simulink model "PPS_Scenario_003_cs"  (Simulink 7.6)
settings: Solver=ode5  SolverMode=SingleTasking  StartTime=0.0  StopTime=inf  FixedStep=1/100  RelTol=1e-3
PreLoadFcn:
  | check_NUTS_defined;
  | 
  | assignin('base',['model_closed_' bdroot],false);
  | 
  | addpath('../includes_PPS');
  | 
  | if exist('PPS_Model_sfun.mexw64')==3
  | delete PPS_Model_sfun.mexw64;
  | end
  | 
  | if exist('PPS_Model_sfun.mexw32') ==3
  | delete PPS_Model_sfun.mexw32;
  | end
  | 
  | switch version('-release')
  | case {'2010a', '2010b', '2011a'}
  | addpath('../includes_PPS/ML2010a');
  | case {'2011b', '2012a', '2012b'}
  | addpath('../includes_PPS/ML2011b');
  | otherwise
  | addpath('../includes_PPS/ML2011b');
  | end
InitFcn:
  | PreScanExperimentInitFcn(bdroot)
StopFcn:
  | PreScanExperimentStopFcn(bdroot)
undefined symbols (not defined in the file): DiscIntNeverNeededParam, InitImageOutputDir, x_ini_VRML, y_ini_VRML, z_ini_VRML
libraries: PreScanSimulinkLibrary x48, simulink x27, PreScanUsefulBlocks x20, simulink_extras x9, simulink_need_slupdate x1
(part 2 of 14)

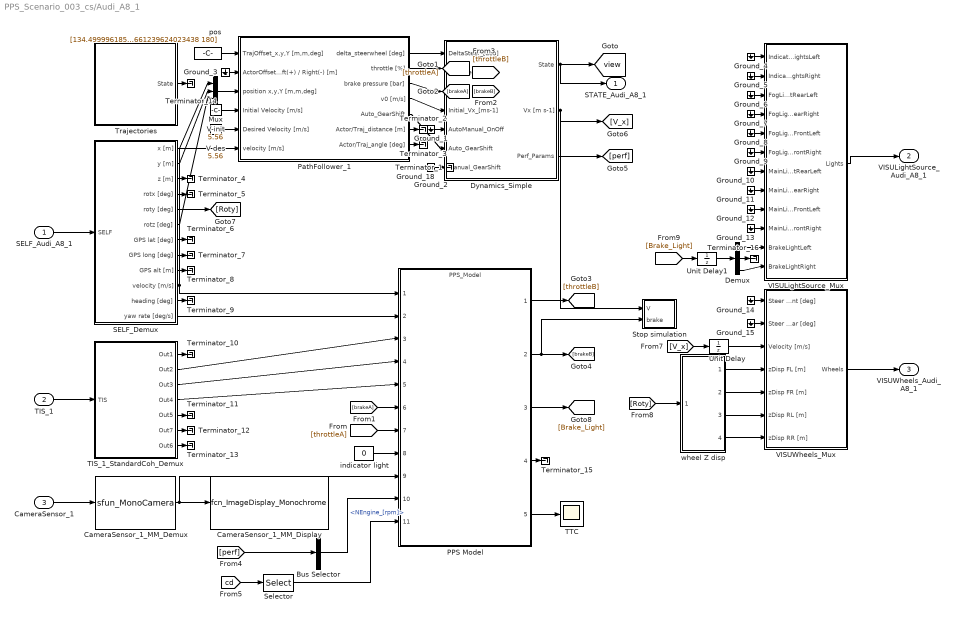
== system PPS_Scenario_003_cs/Audi_A8_1 ==
  SELF_Audi_A8_1 : Inport  Tag=SELFInport
  TIS_1 : Inport  Tag=RadarInport  Port=2  OutDataTypeStr=Bus: PRESCAN_SCANNERSENSORMESSAGE
  CameraSensor_1 : Inport  Tag=CameraSensorInport  Port=3  SampleTime=1/50
  Bus Selector : BusSelector  OutputSignals=NEngine_[rpm]
  CameraSensor_1_MM_Demux : S-Function  Tag=CameraSensor_Monochrome_Demux  FunctionName=sfun_MonoCamera  Parameters=[VerticalResolution HorizontalResolution] FrameRate SensorName CameraType SharedMemTag SharedMemRightTag DataType HasInputPort  EnableBusSupport=off  mask{HorizontalResolution=500, VerticalResolution=375, FrameRate=50, SensorName=CameraSensor_1, CameraType=Mono, SharedMemTag=CameraSensor_1_monoBeam_viewer_RGB, SharedMemRightTag=CameraSensor_1_StereoRight_viewer_RGB, DataType=uint8, HasInputPort=1}
      mask prompts: HorizontalResolution "User Specified: Horizontal Resolution [pixels]"; VerticalResolution "User Specified: Vertical Resolution [pixels]"; FrameRate "User Specified: Frame Rate [Hz]"; SensorName "User Specified: Camera Sensor Name"; CameraType "Camera type"; SharedMemTag "Tag for shared memory for main img"; SharedMemRightTag "Tag for shared memory for right img"; DataType "Image data type"; HasInputPort "Has input port"
      mask init:
      | if CameraType==1
      |     CameraTypeName='MONO';
      |     CameraPort1Name='I';
      |     CameraPort2Name='I';
      |     PortNumber=0;
      | else
      |     CameraTypeName='STEREO';
      |     CameraPort1Name='Left';
      |     CameraPort2Name='Right';
      |     PortNumber=1;
      | end
      settings: DeleteFcn=PreScanBlockDeleteFcn;
      mask StyleString: edit,edit,edit,edit,popup(Mono|Stereo),edit,edit,popup(uint8|single),edit
      mask Display:
      | fprintf('%s CAMERA:\n Monochrome\n%s \n V: %d x %d \n %d fps',CameraTypeName,SensorName,VerticalResolution,HorizontalResolution,FrameRate)
      | port_label('output',1,CameraPort1Name)
      | port_label('output',PortNumber+1,CameraPort2Name)
  CameraSensor_1_MM_Display : M-S-Function  Tag=CameraSensor_Monochrome_Display  InitFcn=InitImageOutputDir(gcb);  FunctionName=fcn_ImageDisplay_Monochrome  Parameters=SensorName EnableDisplay EnablePosition DisplayPosition FigureHandle SaveResults BitmapFormat TempOutputDir CameraType DataType  mask(PreScan Monochrome Display Block){SensorName=CameraSensor_1, EnableDisplay=on, EnablePosition=off, DisplayPosition=[10 10 500 375], FigureHandle=700, SaveResults=off, Format=PNG, TempOutputDir=0, CameraType=Mono, DataType=uint8}
      mask prompts: SensorName "User Specified: Title of Display"; EnableDisplay "Active"; EnablePosition "Set Display window position"; DisplayPosition "Display window position [xpos ypos width height]"; FigureHandle "Unique handle"; SaveResults "Save results"; TempOutputDir "OutputDir"; CameraType "Camera Type"; DataType "Image Data Type"
      mask help: This block displays the Monochrome output of a PreScan camera sensor.
      mask init:
      | if EnableDisplay
      |     EnableString='';
      |     EnableColor='gray';
      | else
      |     EnableString='INACTIVE';
      |     EnableColor='red';
      | end
      | switch Format
      |     case 1
      |         BitmapFormat = 'png';
      |     case 2
      |         BitmapFormat = 'bmp';
      |     case 3
      |         BitmapFormat = 'jpg';
      | end
      | if CameraType==1
      |     CameraTypeName='MONO';
      |     PortNumber=0;
      | else
      |     CameraTypeName='STEREO';
      |     PortNumber=1;
      | end
      settings: CopyFcn=CopyFcnDisplay  DeleteFcn=PreScanBlockDeleteFcn;  ModelCloseFcn=fcn_ImageDisplay_ModelCloseFcn
      mask Help: eval('openHelp(457)')
      mask StyleString: edit,checkbox,checkbox,edit,edit,checkbox,popup(PNG|BMP|JPG),edit,popup(Mono|Stereo),popup(uint8|single)
      mask CallbackString:
      | ||MV=get_param(gcb,'MaskVisibilities');
      | if strcmp(get_param(gcb,'EnablePosition'),'on')
      |     MV{4}='on';
      | else
      |     MV{4}='off';
      | end
      | set_param(gcb,'MaskVisibilities',MV);|||||||
      mask Display:
      | color(EnableColor);
      | fprintf('%s\n DISPLAY:\n Monochrome\n %s',EnableString,SensorName)
      | port_label('input',1,'I')
      | port_label('input',PortNumber+1,'I')
  Demux : Demux  Outputs=3
  Dynamics_Simple : Subsystem  Tag=Simple_Vehicle_Dynamics  mask(PreScan Block: Simple Dynamics){Migrate=off, TimeStep=1/100, ComputationMode=Continuous_Time}
      mask prompts: Migrate "Migrate. During migration this block will be replaced by a newer one."; TimeStep "Auto assigned: Time Step [s]"; ComputationMode "Computation mode:"
      mask help:
      | The Simple Dynamics Model is selected in the GUI to simulate vehicle dynamics behavior.
      |
      | The Simple Dynamics Model is completely open to the user. The parameters of this model can be set in the Simple Dynamics dialog in the GUI.
      |
      | For more information, please click Help.
      mask init:
      | p = SimpleDyn_pars;
      settings: DeleteFcn=PreScanBlockDeleteFcn;
      mask Help: eval('openHelp(220)')
      mask Display:
      | image(imread('SimpleDyn.png'))
      | port_label('input', 1, '{\delta}_S_t_ _e_e_r [deg]','texmode','on')
      | port_label('input', 2, 'Throttle [%]')
      | port_label('input', 3, 'Brake Pres [bar]')
      | port_label('input', 4, 'V_0 [ms-1]','texmode','on')
      | port_label('input', 5, 'Auto=[0]/Manual=[1]')
      | port_label('input', 6, 'Auto_GearShift')
      | port_label('input', 7, 'Manual_GearShift')
      | port_label('output', 1, 'State')
      | port_label('output', 2, 'Vx [ms-1]')
      | port_label('output', 3, 'Perf Params')
  Ground_{1..15,18} (16 alike) : Ground
  Mux : Mux  Inputs=3
  PPS Model : ModelReference  StopFcn=|  ModelNameDialog=PPS_Model  SimulationMode=Normal  ModelReferenceVersion=1.1238  CopyOfModelName=PPS_Model
      | if VRU_DisplaySwitch
      | CSpanel = findobj('Tag','cs_panel');
      | CSvalue = findobj('Tag','cs_value');
      | if VRU_EGO_State_Coll
      |    % Collision occured
      | %	bname = find_system('Tag', 'test num');	% get block name
      | %	test_num = mod( str2num(get_param(bname{:},'Value')), 5 );	% get block value
      | %	vel = ( test_num )*10+10;	% velocity
      |    set(CSpanel, 'BorderWidth',2, 'ForegroundColor',[0 120/255 0], 'HighlightColor',[0 120/255 0], 'ShadowColor', [0 120/255 0]);
      |    set(CSvalue, 'ForegroundColor',[0 120/255 0], 'String', strcat('Speed reduction', sprintf( ' %.1f ',VRU_EGO_State_BrakeVel-VRU_EGO_State_Coll), ' km/h'));
      |    set(CSpanel, 'Visible', 'On');
      |    set(CSvalue, 'Visible', 'On');
      | else
      |     if VRU_EGO_State_Flag06
      |         % Collision almost occur
      | 	set(CSpanel, 'BorderWidth',2, 'ForegroundColor','Green', 'HighlightColor','Green', 'ShadowColor', 'Green');
      | 	set(CSvalue, 'ForegroundColor','Green', 'String', 'Collision avoided');
      |         set(CSpanel, 'Visible', 'On');
      |         set(CSvalue, 'Visible', 'On');
      |     else
      |         % No risk of collision
      | 	set(CSpanel, 'Visible', 'Off');
      |         set(CSvalue, 'Visible', 'Off');
      |     end
      | end
      | clear CSpanel CSvalue VRU_EGO_State_Flag06 VRU_EGO_State_BrakeVel
      | end
      | PPS_Speed_Profile(VRU_simout,VRU_EGO_State_Coll);
      | PPS_TTC_Profile(VRU_simout,VRU_EGO_State_Coll);
  PathFollower_1 : Subsystem  Tag=pathFollower  mask(PreScan Block: Path Follower){Migrate=on, FileName='Car_trajectory_1.mat', TunableSteeringGain=1, XShifting_wrt_COG=0}
      mask prompts: Migrate "Migrate. During migration this block will be replaced by a newer one."; FileName "Trajectory Name"; TunableSteeringGain "TunableSteeringGain [-]"; XShifting_wrt_COG "XShifting_wrt_COG [m]"
      mask help:
      | The Path Follower Model is selected in the GUI to simulate driver behavior.
      |
      | For more information, please click Help.
      mask init:
      | load(['trajectories/',eval(FileName)])
      | traject=trajectory';
      | 
      | Traj_x=traject(:,2);
      | Traj_y=traject(:,3);
      | Traj_z=traject(:,4);
      | Traj_vx=traject(:,8);
      | Traj_vy=traject(:,9);
      | Traj_vz=traject(:,10);
      mask Help: eval('openHelp(232)')
  SELF_Demux : Subsystem  Tag=DemuxSELF
      settings: DeleteFcn=PreScanBlockDeleteFcn;
      mask Type: PreScan Demux Block:
      mask Display:
      | port_label('output',1,'x [m]')
      | port_label('output',2,'y [m]')
      | port_label('output',3,'z [m]','texmode','on')
      | port_label('output',4,'Rotx [deg]','texmode','on')
      | port_label('output',5,'Roty [deg]','texmode','on')
      | port_label('output',6,'Rotz [deg]','texmode','on')
      | port_label('output',7,'GPS lat [deg]','texmode','on')
      | port_label('output',8,'GPS long [deg]','texmode','on')
      | port_label('output',9,'GPS alt [m]','texmode','on')
      | port_label('output',10,'Velocity [m/s]')
      | port_label('output',11,'Heading [deg]')
      | port_label('output',12,'Yaw rate [deg/s]')
  Selector : Selector  InputPortWidth=5  IndexOptions=Index vector (dialog)  Indices=1  OutputSizes=1
  Stop simulation : Subsystem
  TIS_1_StandardCoh_Demux : Subsystem  TreatAsAtomicUnit=on  mask(PreScan Demux Block: TIS){MAXMESSAGES=32}
      mask prompts: MAXMESSAGES "Number of Objects"
      mask Help: eval('openHelp(441)')
      mask Display:
      | port_label('input',1,'TIS')
      | port_label('output',1,'Beam ID [-]')
      | port_label('output',2,'Range [m]')
      | port_label('output',3,'DopplerVelocity [m/s]')
      | port_label('output',4,'{\theta} [deg]','texmode','on')
      | port_label('output',5,'{\phi} [deg]','texmode','on')
      | port_label('output',6,'Target ID [-]','texmode','on')
      | port_label('output',7,'TIS Data','texmode','on')
  TTC : Scope
      settings: TimeRange=4.5  YMin=8  YMax=15
  Terminator_{1..16} (16 alike) : Terminator
  Trajectories : Subsystem  Tag=Trajectories
      settings: DeleteFcn=PreScanBlockDeleteFcn;
      mask Type: PreScan Source Block: Trajectories
      mask Description:
      | The Trajectory block contains the trajectories defined in the PreScan Experiment Editor. The output of the trajectory block is the (vehicle) State.
      | 
      | For more information, please click Help.
      mask Help: eval('openHelp(312)')
      mask Display: image(imread('Trajectory.png'));
  Unit Delay : UnitDelay  SampleTime=-1
  Unit Delay1 : UnitDelay  SampleTime=-1
  V des : Constant  Value=5.56
  V init : Constant  Value=5.56
  VISULightSource_Mux : Subsystem  Tag=MuxLightSource
      settings: DeleteFcn=PreScanBlockDeleteFcn;
      mask Type: PreScan Mux Block:
  VISUWheels_Mux : Subsystem  Tag=MuxWheels  mask(PreScan Mux Block:){TimeStep=1/100}
      mask prompts: TimeStep "Auto Assigned: Time Step [s]"
      settings: DeleteFcn=PreScanBlockDeleteFcn;
  indicator light : Constant  Value=0
  pos : Constant  Tag=pos  Value=[134.49999618530273 66.661239624023438 180]
  wheel Z disp : Subsystem  InitFcn=a = 1.17;  mask{a=1.17, b=1.77}
      mask prompts: a "Distance to the front wheel from cars center of gravity [m]"; b "Distance to the back wheel from cars center of gravity [m]"
      mask help: Simple Dynamics parameters
  STATE_Audi_A8_1 : Outport  Tag=StateOutport
  VISULightSource_Audi_A8_1 : Outport  Tag=VisuLightsOutport  Port=2  SampleTime=1/100
  VISUWheels_Audi_A8_1 : Outport  Tag=VisuWheelsOutport  Port=3  SampleTime=1/100
  tag scope: view=global
  wires:
  PPS Model/1 -> [throttleB]
  PPS Model/2 -> [brakeB], Stop simulation/2(brake)
  [perf] -> Bus Selector/1
  [cd] -> Selector/1
  PPS Model/5 -> TTC/1
  PPS Model/4 -> Terminator_15/1
  [brakeA] -> PPS Model/6
  [throttleA] -> PPS Model/7
  indicator light/1 -> PPS Model/8
  Bus Selector/1 -> PPS Model/10  "<NEngine_[rpm]>"
  Selector/1 -> PPS Model/11
  TIS_1_StandardCoh_Demux/2(Out2) -> PPS Model/3
  TIS_1_StandardCoh_Demux/3(Out3) -> PPS Model/4
  TIS_1_StandardCoh_Demux/4(Out4) -> PPS Model/5
  PPS Model/3 -> [Brake_Light]
  [Roty] -> wheel Z disp/1(rotY [deg])
  [V_x] -> Unit Delay/1
  Unit Delay1/1 -> Demux/1
  [Brake_Light] -> Unit Delay1/1
  Demux/2 -> Terminator_16/1
  pos/1 -> PathFollower_1/1(TrajOffset_x,y,Y [m,m,deg])
  SELF_Audi_A8_1/1 -> SELF_Demux/1(SELF)
  CameraSensor_1/1 -> CameraSensor_1_MM_Demux/1
  VISULightSource_Mux/1(Lights) -> VISULightSource_Audi_A8_1/1
  VISUWheels_Mux/1(Wheels) -> VISUWheels_Audi_A8_1/1
  Dynamics_Simple/2(Vx [m s-1]) -> Stop simulation/1(V), [V_x]
  PathFollower_1/1(delta_steerwheel [deg]) -> Dynamics_Simple/1(DeltaSteer_[deg])
  PathFollower_1/2(throttle [%]) -> [throttleA]
  PathFollower_1/3(brake pressure [bar]) -> [brakeA]
  PathFollower_1/4(v0 [m/s]) -> Dynamics_Simple/4(Initial_Vx_[ms-1])
  PathFollower_1/5(Auto_GearShift) -> Dynamics_Simple/6(Auto_GearShift)
  CameraSensor_1_MM_Demux/1 -> CameraSensor_1_MM_Display/1, PPS Model/9
  Dynamics_Simple/1(State) -> STATE_Audi_A8_1/1, [view]
  TIS_1/1 -> TIS_1_StandardCoh_Demux/1(TIS)
  SELF_Demux/6(rotz [deg]) -> Mux/3
  SELF_Demux/10(velocity [m/s]) -> PathFollower_1/6(velocity [m/s]), PPS Model/1
  SELF_Demux/2(y [m]) -> Mux/2
  SELF_Demux/1(x [m]) -> Mux/1
  Mux/1 -> PathFollower_1/3(position x,y,Y [m,m,deg])
  V init/1 -> PathFollower_1/4(Initial Velocity [m/s])
  SELF_Demux/12(yaw rate [deg/s]) -> PPS Model/2
  wheel Z disp/1(zDisp FL [m]) -> VISUWheels_Mux/4(zDisp FL [m])
  wheel Z disp/2(zDisp FR [m]) -> VISUWheels_Mux/5(zDisp FR [m])
  wheel Z disp/3(zDisp RL [m]) -> VISUWheels_Mux/6(zDisp RL [m])
  wheel Z disp/4(zDisp RR [m]) -> VISUWheels_Mux/7(zDisp RR [m])
  V des/1 -> PathFollower_1/5(Desired Velocity [m/s])
  [throttleB] -> Dynamics_Simple/2(Throttle)
  [brakeB] -> Dynamics_Simple/3(Brake)
  Dynamics_Simple/3(Perf_Params) -> [perf]
  Unit Delay/1 -> VISUWheels_Mux/3(Velocity [m/s])
  Demux/1 -> VISULightSource_Mux/11(BrakeLightLeft)
  Demux/3 -> VISULightSource_Mux/12(BrakeLightRight)
  SELF_Demux/5(roty [deg]) -> [Roty]
  Ground_1/1 -> Dynamics_Simple/5(AutoManual_OnOff)
  Ground_2/1 -> Dynamics_Simple/7(Manual_GearShift)
  Ground_18/1 -> Terminator_1/1
  Ground_3/1 -> PathFollower_1/2(ActorOffset_Left(+) / Right(-) [m])
  PathFollower_1/6(Actor/Traj_distance [m]) -> Terminator_2/1
  PathFollower_1/7(Actor/Traj_angle [deg]) -> Terminator_3/1
  SELF_Demux/3(z [m]) -> Terminator_4/1
  SELF_Demux/4(rotx [deg]) -> Terminator_5/1
  SELF_Demux/7(GPS lat [deg]) -> Terminator_6/1
  SELF_Demux/8(GPS long [deg]) -> Terminator_7/1
  SELF_Demux/9(GPS alt [m]) -> Terminator_8/1
  SELF_Demux/11(heading [deg]) -> Terminator_9/1
  TIS_1_StandardCoh_Demux/1(Out1) -> Terminator_10/1
  TIS_1_StandardCoh_Demux/5(Out5) -> Terminator_11/1
  TIS_1_StandardCoh_Demux/6(Out7) -> Terminator_12/1
  TIS_1_StandardCoh_Demux/7(Out6) -> Terminator_13/1
  Trajectories/1(State) -> Terminator_14/1
  Ground_4/1 -> VISULightSource_Mux/1(IndicatorLightsLeft)
  Ground_5/1 -> VISULightSource_Mux/2(IndicatorLightsRight)
  Ground_6/1 -> VISULightSource_Mux/3(FogLightRearLeft)
  Ground_7/1 -> VISULightSource_Mux/4(FogLightRearRight)
  Ground_8/1 -> VISULightSource_Mux/5(FogLightFrontLeft)
  Ground_9/1 -> VISULightSource_Mux/6(FogLightFrontRight)
  Ground_10/1 -> VISULightSource_Mux/7(MainLightRearLeft)
  Ground_11/1 -> VISULightSource_Mux/8(MainLightRearRight)
  Ground_12/1 -> VISULightSource_Mux/9(MainLightFrontLeft)
  Ground_13/1 -> VISULightSource_Mux/10(MainLightFrontRight)
  Ground_14/1 -> VISUWheels_Mux/1(Steer Angle Front [deg])
  Ground_15/1 -> VISUWheels_Mux/2(Steer Angle Rear [deg])

== system PPS_Scenario_003_cs/BMW_X5_1 ==
  SELF_BMW_X5_1 : Inport  Tag=SELFInport
  Dynamics_Empty : Subsystem  Tag=Dynamics_Empty
      mask Display: port_label('output', 1, 'State');text(0,0,' Empty\n')
  SELF_Demux : Subsystem  Tag=DemuxSELF
      settings: DeleteFcn=PreScanBlockDeleteFcn;
      mask Type: PreScan Demux Block:
      mask Display:
      | port_label('output',1,'x [m]')
      | port_label('output',2,'y [m]')
      | port_label('output',3,'z [m]','texmode','on')
      | port_label('output',4,'Rotx [deg]','texmode','on')
      | port_label('output',5,'Roty [deg]','texmode','on')
      | port_label('output',6,'Rotz [deg]','texmode','on')
      | port_label('output',7,'GPS lat [deg]','texmode','on')
      | port_label('output',8,'GPS long [deg]','texmode','on')
      | port_label('output',9,'GPS alt [m]','texmode','on')
      | port_label('output',10,'Velocity [m/s]')
      | port_label('output',11,'Heading [deg]')
      | port_label('output',12,'Yaw rate [deg/s]')
  Terminator_{1..12} (12 alike) : Terminator
  STATE_BMW_X5_1 : Outport  Tag=StateOutport
  wires:
  SELF_BMW_X5_1/1 -> SELF_Demux/1(SELF)
  Dynamics_Empty/1(State) -> STATE_BMW_X5_1/1
  SELF_Demux/1(x [m]) -> Terminator_1/1
  SELF_Demux/2(y [m]) -> Terminator_2/1
  SELF_Demux/3(z [m]) -> Terminator_3/1
  SELF_Demux/4(rotx [deg]) -> Terminator_4/1
  SELF_Demux/5(roty [deg]) -> Terminator_5/1
  SELF_Demux/6(rotz [deg]) -> Terminator_6/1
  SELF_Demux/7(GPS lat [deg]) -> Terminator_7/1
  SELF_Demux/8(GPS long [deg]) -> Terminator_8/1
  SELF_Demux/9(GPS alt [m]) -> Terminator_9/1
  SELF_Demux/10(velocity [m/s]) -> Terminator_10/1
  SELF_Demux/11(heading [deg]) -> Terminator_11/1
  SELF_Demux/12(yaw rate [deg/s]) -> Terminator_12/1

== system PPS_Scenario_003_cs/BMW_X5_2 ==
  SELF_BMW_X5_2 : Inport  Tag=SELFInport
  Dynamics_Empty : Subsystem  Tag=Dynamics_Empty
      mask Display: port_label('output', 1, 'State');text(0,0,' Empty\n')
  SELF_Demux : Subsystem  Tag=DemuxSELF
      settings: DeleteFcn=PreScanBlockDeleteFcn;
      mask Type: PreScan Demux Block:
      mask Display:
      | port_label('output',1,'x [m]')
      | port_label('output',2,'y [m]')
      | port_label('output',3,'z [m]','texmode','on')
      | port_label('output',4,'Rotx [deg]','texmode','on')
      | port_label('output',5,'Roty [deg]','texmode','on')
      | port_label('output',6,'Rotz [deg]','texmode','on')
      | port_label('output',7,'GPS lat [deg]','texmode','on')
      | port_label('output',8,'GPS long [deg]','texmode','on')
      | port_label('output',9,'GPS alt [m]','texmode','on')
      | port_label('output',10,'Velocity [m/s]')
      | port_label('output',11,'Heading [deg]')
      | port_label('output',12,'Yaw rate [deg/s]')
  Terminator_{1..12} (12 alike) : Terminator
  STATE_BMW_X5_2 : Outport  Tag=StateOutport
  wires:
  SELF_BMW_X5_2/1 -> SELF_Demux/1(SELF)
  Dynamics_Empty/1(State) -> STATE_BMW_X5_2/1
  SELF_Demux/1(x [m]) -> Terminator_1/1
  SELF_Demux/2(y [m]) -> Terminator_2/1
  SELF_Demux/3(z [m]) -> Terminator_3/1
  SELF_Demux/4(rotx [deg]) -> Terminator_4/1
  SELF_Demux/5(roty [deg]) -> Terminator_5/1
  SELF_Demux/6(rotz [deg]) -> Terminator_6/1
  SELF_Demux/7(GPS lat [deg]) -> Terminator_7/1
  SELF_Demux/8(GPS long [deg]) -> Terminator_8/1
  SELF_Demux/9(GPS alt [m]) -> Terminator_9/1
  SELF_Demux/10(velocity [m/s]) -> Terminator_10/1
  SELF_Demux/11(heading [deg]) -> Terminator_11/1
  SELF_Demux/12(yaw rate [deg/s]) -> Terminator_12/1

== system PPS_Scenario_003_cs/BMW_Z3_1 ==
  SELF_BMW_Z3_1 : Inport  Tag=SELFInport
  Dynamics_Empty : Subsystem  Tag=Dynamics_Empty
      mask Display: port_label('output', 1, 'State');text(0,0,' Empty\n')
  SELF_Demux : Subsystem  Tag=DemuxSELF
      settings: DeleteFcn=PreScanBlockDeleteFcn;
      mask Type: PreScan Demux Block:
      mask Display:
      | port_label('output',1,'x [m]')
      | port_label('output',2,'y [m]')
      | port_label('output',3,'z [m]','texmode','on')
      | port_label('output',4,'Rotx [deg]','texmode','on')
      | port_label('output',5,'Roty [deg]','texmode','on')
      | port_label('output',6,'Rotz [deg]','texmode','on')
      | port_label('output',7,'GPS lat [deg]','texmode','on')
      | port_label('output',8,'GPS long [deg]','texmode','on')
      | port_label('output',9,'GPS alt [m]','texmode','on')
      | port_label('output',10,'Velocity [m/s]')
      | port_label('output',11,'Heading [deg]')
      | port_label('output',12,'Yaw rate [deg/s]')
  Terminator_{1..12} (12 alike) : Terminator
  STATE_BMW_Z3_1 : Outport  Tag=StateOutport
  wires:
  SELF_BMW_Z3_1/1 -> SELF_Demux/1(SELF)
  Dynamics_Empty/1(State) -> STATE_BMW_Z3_1/1
  SELF_Demux/1(x [m]) -> Terminator_1/1
  SELF_Demux/2(y [m]) -> Terminator_2/1
  SELF_Demux/3(z [m]) -> Terminator_3/1
  SELF_Demux/4(rotx [deg]) -> Terminator_4/1
  SELF_Demux/5(roty [deg]) -> Terminator_5/1
  SELF_Demux/6(rotz [deg]) -> Terminator_6/1
  SELF_Demux/7(GPS lat [deg]) -> Terminator_7/1
  SELF_Demux/8(GPS long [deg]) -> Terminator_8/1
  SELF_Demux/9(GPS alt [m]) -> Terminator_9/1
  SELF_Demux/10(velocity [m/s]) -> Terminator_10/1
  SELF_Demux/11(heading [deg]) -> Terminator_11/1
  SELF_Demux/12(yaw rate [deg/s]) -> Terminator_12/1

== system PPS_Scenario_003_cs/CameraSensor_1 ==
  Demux : Demux  Outputs=[1 -1]
  Terminator : Terminator
  U1 : Outport
  wires:
  Demux/2 -> Terminator/1
  Demux/1 -> U1/1
  [SimCoreSensors] -> Demux/1

== system PPS_Scenario_003_cs/CarTrailer_SingleAxle_1 ==
  SELF_CarTrailer_SingleAxle_1 : Inport  Tag=SELFInport
  SELF_Demux : Subsystem  Tag=DemuxSELF
      settings: DeleteFcn=PreScanBlockDeleteFcn;
      mask Type: PreScan Demux Block:
      mask Display:
      | port_label('output',1,'x [m]')
      | port_label('output',2,'y [m]')
      | port_label('output',3,'z [m]','texmode','on')
      | port_label('output',4,'Rotx [deg]','texmode','on')
      | port_label('output',5,'Roty [deg]','texmode','on')
      | port_label('output',6,'Rotz [deg]','texmode','on')
      | port_label('output',7,'GPS lat [deg]','texmode','on')
      | port_label('output',8,'GPS long [deg]','texmode','on')
      | port_label('output',9,'GPS alt [m]','texmode','on')
      | port_label('output',10,'Velocity [m/s]')
      | port_label('output',11,'Heading [deg]')
      | port_label('output',12,'Yaw rate [deg/s]')
  Terminator_{1..14} (14 alike) : Terminator
  TrailerConverter : Subsystem  Tag=TrailerConverter  mask(PreScan TrailerConvertor block){e_truck=2.08, D_dolly=0, D_trailer=2.69}
      mask prompts: e_truck "Distance reference point e to coupling"; D_dolly "Distance coupling dolly to axle"; D_trailer "Distance coupling trailer to axle"
      mask help:
      | This block calculates the coordinates and heading
      | of full trailer (container with dolly).
      | As input, rotation point of the truck is given.
      | Coordinates of the towball are calculated
      | based on input parameters.
      mask Help: eval('openHelp(1035)')
      mask Display: image(imread('fullTrailer_Schema.png'))
  TrailerKinematics : Subsystem  Tag=TrailerKinematics  mask(PreScan TrailerKinematics model){e_hitch=0, wheelbase=2.69, alpha_init=0, TimeStep=1/100}
      mask prompts: e_hitch "Offset: Distance from axle to coupling [m] (positive value if hitch is behind axle)"; wheelbase "Length Trailer: from Rear Axle to Front Axle [m] (positive value)"; alpha_init "Initial RELATIVE YawAngle Trailer wrt Truck [deg] (0 deg: Trailer in line with Truck)"; TimeStep "Time Step [s]"
      mask Help: eval('openHelp(1305)')
      mask Display: image(imread('TrailerKinematics.png'));
  STATE_CarTrailer_SingleAxle_1 : Outport  Tag=StateOutport
  wires:
  SELF_CarTrailer_SingleAxle_1/1 -> SELF_Demux/1(SELF)
  [Ford_Fiesta_1_hitch] -> TrailerKinematics/1(DataFromTruck)
  TrailerKinematics/1(Traject_axle) -> TrailerConverter/1(DataFromAxle), TrailerConverter/2(DataFromHitch)
  TrailerConverter/1(Trailer state) -> STATE_CarTrailer_SingleAxle_1/1
  SELF_Demux/1(x [m]) -> Terminator_1/1
  SELF_Demux/2(y [m]) -> Terminator_2/1
  SELF_Demux/3(z [m]) -> Terminator_3/1
  SELF_Demux/4(rotx [deg]) -> Terminator_4/1
  SELF_Demux/5(roty [deg]) -> Terminator_5/1
  SELF_Demux/6(rotz [deg]) -> Terminator_6/1
  SELF_Demux/7(GPS lat [deg]) -> Terminator_7/1
  SELF_Demux/8(GPS long [deg]) -> Terminator_8/1
  SELF_Demux/9(GPS alt [m]) -> Terminator_9/1
  SELF_Demux/10(velocity [m/s]) -> Terminator_10/1
  SELF_Demux/11(heading [deg]) -> Terminator_11/1
  SELF_Demux/12(yaw rate [deg/s]) -> Terminator_12/1
  TrailerConverter/2(visu_RotConnector) -> Terminator_13/1
  TrailerKinematics/2(Traject_hitch) -> Terminator_14/1

== system PPS_Scenario_003_cs/CollisionDetection ==
  Selector : Selector  IndexMode=Zero-based  IndexOptions=Starting index (dialog)  Indices=PortIndex  OutputSizes=PortWidth(1)
  retrieve CollisionDetection signal : Subsystem
  U : Outport
  U1 : Outport  Port=2
  wires:
  retrieve CollisionDetection signal/1(Out) -> U1/1
  [SimCoreSensors] -> Selector/1
  Selector/1 -> retrieve CollisionDetection signal/1(In), U/1

== system PPS_Scenario_003_cs/Fiat_Bravo_1 ==
  SELF_Fiat_Bravo_1 : Inport  Tag=SELFInport
  Dynamics_Empty : Subsystem  Tag=Dynamics_Empty
      mask Display: port_label('output', 1, 'State');text(0,0,' Empty\n')
  SELF_Demux : Subsystem  Tag=DemuxSELF
      settings: DeleteFcn=PreScanBlockDeleteFcn;
      mask Type: PreScan Demux Block:
      mask Display:
      | port_label('output',1,'x [m]')
      | port_label('output',2,'y [m]')
      | port_label('output',3,'z [m]','texmode','on')
      | port_label('output',4,'Rotx [deg]','texmode','on')
      | port_label('output',5,'Roty [deg]','texmode','on')
      | port_label('output',6,'Rotz [deg]','texmode','on')
      | port_label('output',7,'GPS lat [deg]','texmode','on')
      | port_label('output',8,'GPS long [deg]','texmode','on')
      | port_label('output',9,'GPS alt [m]','texmode','on')
      | port_label('output',10,'Velocity [m/s]')
      | port_label('output',11,'Heading [deg]')
      | port_label('output',12,'Yaw rate [deg/s]')
  Terminator_{1..12} (12 alike) : Terminator
  TextureColor : Constant  Tag=TextureColor  Value="[65  105  225]"
  VISUTextureColor_Mux : Subsystem  Tag=MuxSteer
      settings: DeleteFcn=PreScanBlockDeleteFcn;
      mask Type: PreScan Mux Block:
  STATE_Fiat_Bravo_1 : Outport  Tag=StateOutport
  VISUTextureColor_Fiat_Bravo_1 : Outport  Tag=VisuTextureColorOutport  Port=2  SampleTime=1/100
  wires:
  SELF_Fiat_Bravo_1/1 -> SELF_Demux/1(SELF)
  VISUTextureColor_Mux/1(TextureColor) -> VISUTextureColor_Fiat_Bravo_1/1
  TextureColor/1 -> VISUTextureColor_Mux/1(RGB [-,-,-])
  Dynamics_Empty/1(State) -> STATE_Fiat_Bravo_1/1
  SELF_Demux/1(x [m]) -> Terminator_1/1
  SELF_Demux/2(y [m]) -> Terminator_2/1
  SELF_Demux/3(z [m]) -> Terminator_3/1
  SELF_Demux/4(rotx [deg]) -> Terminator_4/1
  SELF_Demux/5(roty [deg]) -> Terminator_5/1
  SELF_Demux/6(rotz [deg]) -> Terminator_6/1
  SELF_Demux/7(GPS lat [deg]) -> Terminator_7/1
  SELF_Demux/8(GPS long [deg]) -> Terminator_8/1
  SELF_Demux/9(GPS alt [m]) -> Terminator_9/1
  SELF_Demux/10(velocity [m/s]) -> Terminator_10/1
  SELF_Demux/11(heading [deg]) -> Terminator_11/1
  SELF_Demux/12(yaw rate [deg/s]) -> Terminator_12/1

== system PPS_Scenario_003_cs/Fiat_Bravo_2 ==
  SELF_Fiat_Bravo_2 : Inport  Tag=SELFInport
  Dynamics_Empty : Subsystem  Tag=Dynamics_Empty
      mask Display: port_label('output', 1, 'State');text(0,0,' Empty\n')
  SELF_Demux : Subsystem  Tag=DemuxSELF
      settings: DeleteFcn=PreScanBlockDeleteFcn;
      mask Type: PreScan Demux Block:
      mask Display:
      | port_label('output',1,'x [m]')
      | port_label('output',2,'y [m]')
      | port_label('output',3,'z [m]','texmode','on')
      | port_label('output',4,'Rotx [deg]','texmode','on')
      | port_label('output',5,'Roty [deg]','texmode','on')
      | port_label('output',6,'Rotz [deg]','texmode','on')
      | port_label('output',7,'GPS lat [deg]','texmode','on')
      | port_label('output',8,'GPS long [deg]','texmode','on')
      | port_label('output',9,'GPS alt [m]','texmode','on')
      | port_label('output',10,'Velocity [m/s]')
      | port_label('output',11,'Heading [deg]')
      | port_label('output',12,'Yaw rate [deg/s]')
  Terminator_{1..12} (12 alike) : Terminator
  STATE_Fiat_Bravo_2 : Outport  Tag=StateOutport
  wires:
  SELF_Fiat_Bravo_2/1 -> SELF_Demux/1(SELF)
  Dynamics_Empty/1(State) -> STATE_Fiat_Bravo_2/1
  SELF_Demux/1(x [m]) -> Terminator_1/1
  SELF_Demux/2(y [m]) -> Terminator_2/1
  SELF_Demux/3(z [m]) -> Terminator_3/1
  SELF_Demux/4(rotx [deg]) -> Terminator_4/1
  SELF_Demux/5(roty [deg]) -> Terminator_5/1
  SELF_Demux/6(rotz [deg]) -> Terminator_6/1
  SELF_Demux/7(GPS lat [deg]) -> Terminator_7/1
  SELF_Demux/8(GPS long [deg]) -> Terminator_8/1
  SELF_Demux/9(GPS alt [m]) -> Terminator_9/1
  SELF_Demux/10(velocity [m/s]) -> Terminator_10/1
  SELF_Demux/11(heading [deg]) -> Terminator_11/1
  SELF_Demux/12(yaw rate [deg/s]) -> Terminator_12/1

== system PPS_Scenario_003_cs/Ford_Fiesta_1 ==
  SELF_Ford_Fiesta_1 : Inport  Tag=SELFInport
  Ground_{1..6} (6 alike) : Ground
  SELF_Demux : Subsystem  Tag=DemuxSELF
      settings: DeleteFcn=PreScanBlockDeleteFcn;
      mask Type: PreScan Demux Block:
      mask Display:
      | port_label('output',1,'x [m]')
      | port_label('output',2,'y [m]')
      | port_label('output',3,'z [m]','texmode','on')
      | port_label('output',4,'Rotx [deg]','texmode','on')
      | port_label('output',5,'Roty [deg]','texmode','on')
      | port_label('output',6,'Rotz [deg]','texmode','on')
      | port_label('output',7,'GPS lat [deg]','texmode','on')
      | port_label('output',8,'GPS long [deg]','texmode','on')
      | port_label('output',9,'GPS alt [m]','texmode','on')
      | port_label('output',10,'Velocity [m/s]')
      | port_label('output',11,'Heading [deg]')
      | port_label('output',12,'Yaw rate [deg/s]')
  Terminator_{1..11} (11 alike) : Terminator
  Trajectories : Subsystem  Tag=Trajectories
      settings: DeleteFcn=PreScanBlockDeleteFcn;
      mask Type: PreScan Source Block: Trajectories
      mask Description:
      | The Trajectory block contains the trajectories defined in the PreScan Experiment Editor. The output of the trajectory block is the (vehicle) State.
      | 
      | For more information, please click Help.
      mask Help: eval('openHelp(312)')
      mask Display: image(imread('Trajectory.png'));
  TruckModel : Subsystem  Tag=TruckModel  mask(PreScan TruckModel Block){wheelbase=0, rear_hitch=0.6, rear_cog=1.48, TimeStep=1/100}
      mask prompts: wheelbase "Wheelbase [m]"; rear_hitch "Rear axle to hitch [m]"; rear_cog "Rear axle to COG [m]"; TimeStep "Time Step [s]"
      mask help:
      | Truck model
      |
      | For more information, please click Help.
      mask init:
      | alpha_init=0;
      | if (rear_cog == 0)
      |      error('TruckModel:rear_cog', 'The distance between the rear_axle and COG must be positive. Change the location of the COG.')
      | end
      mask Help: eval('openHelp(1305)')
      mask Display: image(imread('fullTrailer_Schema.png'))
  VISUWheels_Mux : Subsystem  Tag=MuxWheels  mask(PreScan Mux Block:){TimeStep=1/100}
      mask prompts: TimeStep "Auto Assigned: Time Step [s]"
      settings: DeleteFcn=PreScanBlockDeleteFcn;
  STATE_Ford_Fiesta_1 : Outport  Tag=StateOutport
  VISUWheels_Ford_Fiesta_1 : Outport  Tag=VisuWheelsOutport  Port=2  SampleTime=1/100
  tag scope: Ford_Fiesta_1_hitch=global
  wires:
  SELF_Ford_Fiesta_1/1 -> SELF_Demux/1(SELF)
  VISUWheels_Mux/1(Wheels) -> VISUWheels_Ford_Fiesta_1/1
  TruckModel/1(Out1) -> STATE_Ford_Fiesta_1/1
  Trajectories/1(State) -> TruckModel/1(In1)
  TruckModel/2(DataFromTruck) -> [Ford_Fiesta_1_hitch]
  SELF_Demux/10(velocity [m/s]) -> VISUWheels_Mux/3(Velocity [m/s])
  SELF_Demux/1(x [m]) -> Terminator_1/1
  SELF_Demux/2(y [m]) -> Terminator_2/1
  SELF_Demux/3(z [m]) -> Terminator_3/1
  SELF_Demux/4(rotx [deg]) -> Terminator_4/1
  SELF_Demux/5(roty [deg]) -> Terminator_5/1
  SELF_Demux/6(rotz [deg]) -> Terminator_6/1
  SELF_Demux/7(GPS lat [deg]) -> Terminator_7/1
  SELF_Demux/8(GPS long [deg]) -> Terminator_8/1
  SELF_Demux/9(GPS alt [m]) -> Terminator_9/1
  SELF_Demux/11(heading [deg]) -> Terminator_10/1
  SELF_Demux/12(yaw rate [deg/s]) -> Terminator_11/1
  Ground_1/1 -> VISUWheels_Mux/1(Steer Angle Front [deg])
  Ground_2/1 -> VISUWheels_Mux/2(Steer Angle Rear [deg])
  Ground_3/1 -> VISUWheels_Mux/4(zDisp FL [m])
  Ground_4/1 -> VISUWheels_Mux/5(zDisp FR [m])
  Ground_5/1 -> VISUWheels_Mux/6(zDisp RL [m])
  Ground_6/1 -> VISUWheels_Mux/7(zDisp RR [m])

== system PPS_Scenario_003_cs/GetSensors ==
  dummy : Inport
  GetSensors : M-S-Function  FunctionName=GetSensorsBlock  Parameters=TimeStep NrOfSensors
  tag scope: SimCoreSensors=global
  wires:
  GetSensors/1 -> [SimCoreSensors]
  dummy/1 -> GetSensors/1

== system PPS_Scenario_003_cs/HumanAnimated_1 ==
  SELF_HumanAnimated_1 : Inport  Tag=SELFInport
  Gain : Gain  Gain=[1 1 1 1 1 1 0 0 1]
  SELF_Demux : Subsystem  Tag=DemuxSELF
      settings: DeleteFcn=PreScanBlockDeleteFcn;
      mask Type: PreScan Demux Block:
      mask Display:
      | port_label('output',1,'x [m]')
      | port_label('output',2,'y [m]')
      | port_label('output',3,'z [m]','texmode','on')
      | port_label('output',4,'Rotx [deg]','texmode','on')
      | port_label('output',5,'Roty [deg]','texmode','on')
      | port_label('output',6,'Rotz [deg]','texmode','on')
      | port_label('output',7,'GPS lat [deg]','texmode','on')
      | port_label('output',8,'GPS long [deg]','texmode','on')
      | port_label('output',9,'GPS alt [m]','texmode','on')
      | port_label('output',10,'Velocity [m/s]')
      | port_label('output',11,'Heading [deg]')
      | port_label('output',12,'Yaw rate [deg/s]')
  Terminator_{1..12} (12 alike) : Terminator
  Trajectories : Subsystem  Tag=Trajectories
      settings: DeleteFcn=PreScanBlockDeleteFcn;
      mask Type: PreScan Source Block: Trajectories
      mask Description:
      | The Trajectory block contains the trajectories defined in the PreScan Experiment Editor. The output of the trajectory block is the (vehicle) State.
      | 
      | For more information, please click Help.
      mask Help: eval('openHelp(312)')
      mask Display: image(imread('Trajectory.png'));
  STATE_HumanAnimated_1 : Outport  Tag=StateOutport
  wires:
  SELF_HumanAnimated_1/1 -> SELF_Demux/1(SELF)
  Gain/1 -> STATE_HumanAnimated_1/1
  Trajectories/1(State) -> Gain/1
  SELF_Demux/1(x [m]) -> Terminator_1/1
  SELF_Demux/2(y [m]) -> Terminator_2/1
  SELF_Demux/3(z [m]) -> Terminator_3/1
  SELF_Demux/4(rotx [deg]) -> Terminator_4/1
  SELF_Demux/5(roty [deg]) -> Terminator_5/1
  SELF_Demux/6(rotz [deg]) -> Terminator_6/1
  SELF_Demux/7(GPS lat [deg]) -> Terminator_7/1
  SELF_Demux/8(GPS long [deg]) -> Terminator_8/1
  SELF_Demux/9(GPS alt [m]) -> Terminator_9/1
  SELF_Demux/10(velocity [m/s]) -> Terminator_10/1
  SELF_Demux/11(heading [deg]) -> Terminator_11/1
  SELF_Demux/12(yaw rate [deg/s]) -> Terminator_12/1

== system PPS_Scenario_003_cs/Lightpost_1 ==

== system PPS_Scenario_003_cs/Lightpost_10 ==

== system PPS_Scenario_003_cs/Lightpost_11 ==

== system PPS_Scenario_003_cs/Lightpost_12 ==

== system PPS_Scenario_003_cs/Lightpost_13 ==

== system PPS_Scenario_003_cs/Lightpost_14 ==

== system PPS_Scenario_003_cs/Lightpost_15 ==

== system PPS_Scenario_003_cs/Lightpost_16 ==

== system PPS_Scenario_003_cs/Lightpost_17 ==

== system PPS_Scenario_003_cs/Lightpost_18 ==

== system PPS_Scenario_003_cs/Lightpost_19 ==

== system PPS_Scenario_003_cs/Lightpost_2 ==

== system PPS_Scenario_003_cs/Lightpost_20 ==

== system PPS_Scenario_003_cs/Lightpost_3 ==

== system PPS_Scenario_003_cs/Lightpost_4 ==

== system PPS_Scenario_003_cs/Lightpost_5 ==

== system PPS_Scenario_003_cs/Lightpost_6 ==

== system PPS_Scenario_003_cs/Lightpost_7 ==

== system PPS_Scenario_003_cs/Lightpost_8 ==

== system PPS_Scenario_003_cs/Lightpost_9 ==

== system PPS_Scenario_003_cs/Mazda_RX8_2 ==
  SELF_Mazda_RX8_2 : Inport  Tag=SELFInport
  Dynamics_Empty : Subsystem  Tag=Dynamics_Empty
      mask Display: port_label('output', 1, 'State');text(0,0,' Empty\n')
  SELF_Demux : Subsystem  Tag=DemuxSELF
      settings: DeleteFcn=PreScanBlockDeleteFcn;
      mask Type: PreScan Demux Block:
      mask Display:
      | port_label('output',1,'x [m]')
      | port_label('output',2,'y [m]')
      | port_label('output',3,'z [m]','texmode','on')
      | port_label('output',4,'Rotx [deg]','texmode','on')
      | port_label('output',5,'Roty [deg]','texmode','on')
      | port_label('output',6,'Rotz [deg]','texmode','on')
      | port_label('output',7,'GPS lat [deg]','texmode','on')
      | port_label('output',8,'GPS long [deg]','texmode','on')
      | port_label('output',9,'GPS alt [m]','texmode','on')
      | port_label('output',10,'Velocity [m/s]')
      | port_label('output',11,'Heading [deg]')
      | port_label('output',12,'Yaw rate [deg/s]')
  Terminator_{1..12} (12 alike) : Terminator
  STATE_Mazda_RX8_2 : Outport  Tag=StateOutport
  wires:
  SELF_Mazda_RX8_2/1 -> SELF_Demux/1(SELF)
  Dynamics_Empty/1(State) -> STATE_Mazda_RX8_2/1
  SELF_Demux/1(x [m]) -> Terminator_1/1
  SELF_Demux/2(y [m]) -> Terminator_2/1
  SELF_Demux/3(z [m]) -> Terminator_3/1
  SELF_Demux/4(rotx [deg]) -> Terminator_4/1
  SELF_Demux/5(roty [deg]) -> Terminator_5/1
  SELF_Demux/6(rotz [deg]) -> Terminator_6/1
  SELF_Demux/7(GPS lat [deg]) -> Terminator_7/1
  SELF_Demux/8(GPS long [deg]) -> Terminator_8/1
  SELF_Demux/9(GPS alt [m]) -> Terminator_9/1
  SELF_Demux/10(velocity [m/s]) -> Terminator_10/1
  SELF_Demux/11(heading [deg]) -> Terminator_11/1
  SELF_Demux/12(yaw rate [deg/s]) -> Terminator_12/1

== system PPS_Scenario_003_cs/Mazda_RX8_3 ==
  SELF_Mazda_RX8_3 : Inport  Tag=SELFInport
  Dynamics_Empty : Subsystem  Tag=Dynamics_Empty
      mask Display: port_label('output', 1, 'State');text(0,0,' Empty\n')
  SELF_Demux : Subsystem  Tag=DemuxSELF
      settings: DeleteFcn=PreScanBlockDeleteFcn;
      mask Type: PreScan Demux Block:
      mask Display:
      | port_label('output',1,'x [m]')
      | port_label('output',2,'y [m]')
      | port_label('output',3,'z [m]','texmode','on')
      | port_label('output',4,'Rotx [deg]','texmode','on')
      | port_label('output',5,'Roty [deg]','texmode','on')
      | port_label('output',6,'Rotz [deg]','texmode','on')
      | port_label('output',7,'GPS lat [deg]','texmode','on')
      | port_label('output',8,'GPS long [deg]','texmode','on')
      | port_label('output',9,'GPS alt [m]','texmode','on')
      | port_label('output',10,'Velocity [m/s]')
      | port_label('output',11,'Heading [deg]')
      | port_label('output',12,'Yaw rate [deg/s]')
  Terminator_{1..12} (12 alike) : Terminator
  STATE_Mazda_RX8_3 : Outport  Tag=StateOutport
  wires:
  SELF_Mazda_RX8_3/1 -> SELF_Demux/1(SELF)
  Dynamics_Empty/1(State) -> STATE_Mazda_RX8_3/1
  SELF_Demux/1(x [m]) -> Terminator_1/1
  SELF_Demux/2(y [m]) -> Terminator_2/1
  SELF_Demux/3(z [m]) -> Terminator_3/1
  SELF_Demux/4(rotx [deg]) -> Terminator_4/1
  SELF_Demux/5(roty [deg]) -> Terminator_5/1
  SELF_Demux/6(rotz [deg]) -> Terminator_6/1
  SELF_Demux/7(GPS lat [deg]) -> Terminator_7/1
  SELF_Demux/8(GPS long [deg]) -> Terminator_8/1
  SELF_Demux/9(GPS alt [m]) -> Terminator_9/1
  SELF_Demux/10(velocity [m/s]) -> Terminator_10/1
  SELF_Demux/11(heading [deg]) -> Terminator_11/1
  SELF_Demux/12(yaw rate [deg/s]) -> Terminator_12/1

== system PPS_Scenario_003_cs/Nissan_Cabstar_1 ==
  SELF_Nissan_Cabstar_1 : Inport  Tag=SELFInport
  Dynamics_Empty : Subsystem  Tag=Dynamics_Empty
      mask Display: port_label('output', 1, 'State');text(0,0,' Empty\n')
  SELF_Demux : Subsystem  Tag=DemuxSELF
      settings: DeleteFcn=PreScanBlockDeleteFcn;
      mask Type: PreScan Demux Block:
      mask Display:
      | port_label('output',1,'x [m]')
      | port_label('output',2,'y [m]')
      | port_label('output',3,'z [m]','texmode','on')
      | port_label('output',4,'Rotx [deg]','texmode','on')
      | port_label('output',5,'Roty [deg]','texmode','on')
      | port_label('output',6,'Rotz [deg]','texmode','on')
      | port_label('output',7,'GPS lat [deg]','texmode','on')
      | port_label('output',8,'GPS long [deg]','texmode','on')
      | port_label('output',9,'GPS alt [m]','texmode','on')
      | port_label('output',10,'Velocity [m/s]')
      | port_label('output',11,'Heading [deg]')
      | port_label('output',12,'Yaw rate [deg/s]')
  Terminator_{1..12} (12 alike) : Terminator
  STATE_Nissan_Cabstar_1 : Outport  Tag=StateOutport
  wires:
  SELF_Nissan_Cabstar_1/1 -> SELF_Demux/1(SELF)
  Dynamics_Empty/1(State) -> STATE_Nissan_Cabstar_1/1
  SELF_Demux/1(x [m]) -> Terminator_1/1
  SELF_Demux/2(y [m]) -> Terminator_2/1
  SELF_Demux/3(z [m]) -> Terminator_3/1
  SELF_Demux/4(rotx [deg]) -> Terminator_4/1
  SELF_Demux/5(roty [deg]) -> Terminator_5/1
  SELF_Demux/6(rotz [deg]) -> Terminator_6/1
  SELF_Demux/7(GPS lat [deg]) -> Terminator_7/1
  SELF_Demux/8(GPS long [deg]) -> Terminator_8/1
  SELF_Demux/9(GPS alt [m]) -> Terminator_9/1
  SELF_Demux/10(velocity [m/s]) -> Terminator_10/1
  SELF_Demux/11(heading [deg]) -> Terminator_11/1
  SELF_Demux/12(yaw rate [deg/s]) -> Terminator_12/1

== system PPS_Scenario_003_cs/Nissan_Cabstar_2 ==
  SELF_Nissan_Cabstar_2 : Inport  Tag=SELFInport
  Dynamics_Empty : Subsystem  Tag=Dynamics_Empty
      mask Display: port_label('output', 1, 'State');text(0,0,' Empty\n')
  SELF_Demux : Subsystem  Tag=DemuxSELF
      settings: DeleteFcn=PreScanBlockDeleteFcn;
      mask Type: PreScan Demux Block:
      mask Display:
      | port_label('output',1,'x [m]')
      | port_label('output',2,'y [m]')
      | port_label('output',3,'z [m]','texmode','on')
      | port_label('output',4,'Rotx [deg]','texmode','on')
      | port_label('output',5,'Roty [deg]','texmode','on')
      | port_label('output',6,'Rotz [deg]','texmode','on')
      | port_label('output',7,'GPS lat [deg]','texmode','on')
      | port_label('output',8,'GPS long [deg]','texmode','on')
      | port_label('output',9,'GPS alt [m]','texmode','on')
      | port_label('output',10,'Velocity [m/s]')
      | port_label('output',11,'Heading [deg]')
      | port_label('output',12,'Yaw rate [deg/s]')
  Terminator_{1..12} (12 alike) : Terminator
  STATE_Nissan_Cabstar_2 : Outport  Tag=StateOutport
  wires:
  SELF_Nissan_Cabstar_2/1 -> SELF_Demux/1(SELF)
  Dynamics_Empty/1(State) -> STATE_Nissan_Cabstar_2/1
  SELF_Demux/1(x [m]) -> Terminator_1/1
  SELF_Demux/2(y [m]) -> Terminator_2/1
  SELF_Demux/3(z [m]) -> Terminator_3/1
  SELF_Demux/4(rotx [deg]) -> Terminator_4/1
  SELF_Demux/5(roty [deg]) -> Terminator_5/1
  SELF_Demux/6(rotz [deg]) -> Terminator_6/1
  SELF_Demux/7(GPS lat [deg]) -> Terminator_7/1
  SELF_Demux/8(GPS long [deg]) -> Terminator_8/1
  SELF_Demux/9(GPS alt [m]) -> Terminator_9/1
  SELF_Demux/10(velocity [m/s]) -> Terminator_10/1
  SELF_Demux/11(heading [deg]) -> Terminator_11/1
  SELF_Demux/12(yaw rate [deg/s]) -> Terminator_12/1

== system PPS_Scenario_003_cs/SELF_Audi_A8_1 ==
  Selector : Selector  IndexMode=Zero-based  IndexOptions=Starting index (dialog)  Indices=PortIndex  OutputSizes=PortWidth(1)
  U : Outport
  wires:
  Selector/1 -> U/1
  [SimCoreSensors] -> Selector/1

== system PPS_Scenario_003_cs/SELF_BMW_X5_1 ==
  Selector : Selector  IndexMode=Zero-based  IndexOptions=Starting index (dialog)  Indices=PortIndex  OutputSizes=PortWidth(1)
  U : Outport
  wires:
  Selector/1 -> U/1
  [SimCoreSensors] -> Selector/1

== system PPS_Scenario_003_cs/SELF_BMW_X5_2 ==
  Selector : Selector  IndexMode=Zero-based  IndexOptions=Starting index (dialog)  Indices=PortIndex  OutputSizes=PortWidth(1)
  U : Outport
  wires:
  Selector/1 -> U/1
  [SimCoreSensors] -> Selector/1

== system PPS_Scenario_003_cs/SELF_BMW_Z3_1 ==
  Selector : Selector  IndexMode=Zero-based  IndexOptions=Starting index (dialog)  Indices=PortIndex  OutputSizes=PortWidth(1)
  U : Outport
  wires:
  Selector/1 -> U/1
  [SimCoreSensors] -> Selector/1

== system PPS_Scenario_003_cs/SELF_CarTrailer_SingleAxle_1 ==
  Selector : Selector  IndexMode=Zero-based  IndexOptions=Starting index (dialog)  Indices=PortIndex  OutputSizes=PortWidth(1)
  U : Outport
  wires:
  Selector/1 -> U/1
  [SimCoreSensors] -> Selector/1

== system PPS_Scenario_003_cs/SELF_Fiat_Bravo_1 ==
  Selector : Selector  IndexMode=Zero-based  IndexOptions=Starting index (dialog)  Indices=PortIndex  OutputSizes=PortWidth(1)
  U : Outport
  wires:
  Selector/1 -> U/1
  [SimCoreSensors] -> Selector/1

== system PPS_Scenario_003_cs/SELF_Fiat_Bravo_2 ==
  Selector : Selector  IndexMode=Zero-based  IndexOptions=Starting index (dialog)  Indices=PortIndex  OutputSizes=PortWidth(1)
  U : Outport
  wires:
  Selector/1 -> U/1
  [SimCoreSensors] -> Selector/1

== system PPS_Scenario_003_cs/SELF_Ford_Fiesta_1 ==
  Selector : Selector  IndexMode=Zero-based  IndexOptions=Starting index (dialog)  Indices=PortIndex  OutputSizes=PortWidth(1)
  U : Outport
  wires:
  Selector/1 -> U/1
  [SimCoreSensors] -> Selector/1

== system PPS_Scenario_003_cs/SELF_HumanAnimated_1 ==
  Selector : Selector  IndexMode=Zero-based  IndexOptions=Starting index (dialog)  Indices=PortIndex  OutputSizes=PortWidth(1)
  U : Outport
  wires:
  Selector/1 -> U/1
  [SimCoreSensors] -> Selector/1

== system PPS_Scenario_003_cs/SELF_Mazda_RX8_2 ==
  Selector : Selector  IndexMode=Zero-based  IndexOptions=Starting index (dialog)  Indices=PortIndex  OutputSizes=PortWidth(1)
  U : Outport
  wires:
  Selector/1 -> U/1
  [SimCoreSensors] -> Selector/1

== system PPS_Scenario_003_cs/SELF_Mazda_RX8_3 ==
  Selector : Selector  IndexMode=Zero-based  IndexOptions=Starting index (dialog)  Indices=PortIndex  OutputSizes=PortWidth(1)
  U : Outport
  wires:
  Selector/1 -> U/1
  [SimCoreSensors] -> Selector/1

== system PPS_Scenario_003_cs/SELF_Nissan_Cabstar_1 ==
  Selector : Selector  IndexMode=Zero-based  IndexOptions=Starting index (dialog)  Indices=PortIndex  OutputSizes=PortWidth(1)
  U : Outport
  wires:
  Selector/1 -> U/1
  [SimCoreSensors] -> Selector/1

== system PPS_Scenario_003_cs/SELF_Nissan_Cabstar_2 ==
  Selector : Selector  IndexMode=Zero-based  IndexOptions=Starting index (dialog)  Indices=PortIndex  OutputSizes=PortWidth(1)
  U : Outport
  wires:
  Selector/1 -> U/1
  [SimCoreSensors] -> Selector/1

== system PPS_Scenario_003_cs/SELF_Sphere_1 ==
  Selector : Selector  IndexMode=Zero-based  IndexOptions=Starting index (dialog)  Indices=PortIndex  OutputSizes=PortWidth(1)
  U : Outport
  wires:
  Selector/1 -> U/1
  [SimCoreSensors] -> Selector/1

== system PPS_Scenario_003_cs/SELF_Toyota_Previa_1 ==
  Selector : Selector  IndexMode=Zero-based  IndexOptions=Starting index (dialog)  Indices=PortIndex  OutputSizes=PortWidth(1)
  U : Outport
  wires:
  Selector/1 -> U/1
  [SimCoreSensors] -> Selector/1

== system PPS_Scenario_003_cs/SELF_Toyota_Previa_2 ==
  Selector : Selector  IndexMode=Zero-based  IndexOptions=Starting index (dialog)  Indices=PortIndex  OutputSizes=PortWidth(1)
  U : Outport
  wires:
  Selector/1 -> U/1
  [SimCoreSensors] -> Selector/1

== system PPS_Scenario_003_cs/SELF_Toyota_Previa_3 ==
  Selector : Selector  IndexMode=Zero-based  IndexOptions=Starting index (dialog)  Indices=PortIndex  OutputSizes=PortWidth(1)
  U : Outport
  wires:
  Selector/1 -> U/1
  [SimCoreSensors] -> Selector/1

== system PPS_Scenario_003_cs/SELF_Toyota_Previa_4 ==
  Selector : Selector  IndexMode=Zero-based  IndexOptions=Starting index (dialog)  Indices=PortIndex  OutputSizes=PortWidth(1)
  U : Outport
  wires:
  Selector/1 -> U/1
  [SimCoreSensors] -> Selector/1

== system PPS_Scenario_003_cs/SELF_Toyota_Yaris_1 ==
  Selector : Selector  IndexMode=Zero-based  IndexOptions=Starting index (dialog)  Indices=PortIndex  OutputSizes=PortWidth(1)
  U : Outport
  wires:
  Selector/1 -> U/1
  [SimCoreSensors] -> Selector/1
